simulink model "mainV02_43"  (R2016b)
settings: Solver=FixedStepAuto  StartTime=0.0  StopTime=inf  FixedStep=Ts  MaxStep=0.2  RelTol=1e-2
undefined symbols (not defined in the file): checks, decyear, deltae_degrees, deltafl_degrees, deltafr_degrees, deltar_degrees, deltat_1, deltat_2, deltat_3, deltat_4, deltat_5, Earth, F, ft, groundReaction, initDate, initialValues, LD, leapyear, Light, m, MIL, Newton, Raphson, s, sigbuilder_block, Ts, Vehicle, WGS84
libraries: simulink x21, aerolibutil x19, aerolibtransform2 x9, aerolib6dofsys x5, aerolibasang x4, aerolib6dof2 x4, aerolibwind2 x3, aerolibbdyn x3, aerolibconvert2 x3, aerolibactuator x2, aerolibgravity2 x2, aerolibnav x2
(part 3 of 6)

== system mainV02_43/LIBIS Plant/Custom Variable Mass 6DOF (Euler Angles) (propio) ==
  Forces : Inport  Unit=N  PortDimensions=3
  Moments : Inport  Port=2  Unit=N*m  PortDimensions=3
  m_dot : Inport  Port=3  Unit=kg/s
  mass : Inport  Port=4  Unit=kg
  I_dot : Inport  Port=5  Unit=kg*m^2/s  PortDimensions=[3 3]
  I : Inport  Port=6  Unit=kg*m^2  PortDimensions=[3 3]
  Vre : Inport  Port=7  Unit=m/s
  Calculate DCM & Euler Angles : aerolib6dofsys/DCM & Euler Angles (Euler)  SystemSampleTime=-1
  Calculate omega_dot : aerolib6dofsys/Calculate omega_dot  SystemSampleTime=-1
  "Determine Force, Mass & Inertia" : aerolib6dofsys/Mass & Inertia (custom)  SystemSampleTime=-1
  Disallow CGS : UnitConfiguration  UnitSystemsStr=English,SI,SI (extended)  AllowAllUnitSystems=off
  Out9 : Terminator
  Product : Product  Inputs=*/  SaturateOnIntegerOverflow=on  OutDataTypeStr=Inherit: Same as first input
  Reshape : Reshape  OutputDimensions=""
  Sum2 : Sum  Inputs=|++  SaturateOnIntegerOverflow=on
  Transpose : Math  Operator=transpose  SaturateOnIntegerOverflow=on
  Vbxw : aerolibutil/3x3 Cross Product
  Velocity Conversion : aerolib6dof2/6DOF (Euler Angles)/Velocity Conversion
  Velocity Conversion1 : aerolib6dof2/6DOF (Euler Angles)/Velocity Conversion1
  Velocity Conversion2 : aerolib6dof2/6DOF (Euler Angles)/Velocity Conversion2
  "p,q,r " : Integrator  InitialCondition=pm_0
  "transform to Inertial axes " : aerolib6dof2/6DOF (Euler Angles)/transform to Inertial axes   SystemSampleTime=-1
  ub,vb,wb : Integrator  InitialCondition=Vm_0
  xe,ye,ze : Integrator  InitialCondition=xme_0  UpperSaturationLimit=[inf, inf, initialValues.href]  LowerSaturationLimit=[-inf, -inf, -inf]
  Ve : Outport  Unit=m/s
  Xe : Outport  Port=2  Unit=m
  Euler : Outport  Port=3  Unit=rad
  DCM : Outport  Port=4  Unit=1
  Vb : Outport  Port=5  Unit=m/s
  p,q,r : Outport  Port=6  Unit=rad/s
  pdot,qdot,rdot : Outport  Port=7  Unit=rad/s^2
  Ab : Outport  Port=8  Unit=m/s^2  PortDimensions=3
  wires:
  Velocity Conversion1/1 -> Ve/1
  "Determine Force, Mass & Inertia"/2 -> Product/2
  Vre/1 -> Velocity Conversion2/1
  Calculate DCM & Euler Angles/1 -> DCM/1, Transpose/1
  Transpose/1 -> "transform to Inertial axes "/2
  Calculate DCM & Euler Angles/2 -> Euler/1
  "Determine Force, Mass & Inertia"/4 -> Out9/1
  "p,q,r "/1 -> Calculate DCM & Euler Angles/1, p,q,r/1, Vbxw/2, Calculate omega_dot/1
  xe,ye,ze/1 -> Xe/1
  Velocity Conversion/1 -> Vb/1
  I_dot/1 -> "Determine Force, Mass & Inertia"/6
  "transform to Inertial axes "/1 -> Velocity Conversion1/1, xe,ye,ze/1
  mass/1 -> "Determine Force, Mass & Inertia"/3
  Velocity Conversion2/1 -> "Determine Force, Mass & Inertia"/1
  "Determine Force, Mass & Inertia"/1 -> Product/1
  Forces/1 -> "Determine Force, Mass & Inertia"/2
  Moments/1 -> Calculate omega_dot/3
  Product/1 -> Sum2/1
  m_dot/1 -> "Determine Force, Mass & Inertia"/4
  ub,vb,wb/1 -> Vbxw/1, "transform to Inertial axes "/1, Velocity Conversion/1
  "Determine Force, Mass & Inertia"/3 -> Calculate omega_dot/2
  I/1 -> "Determine Force, Mass & Inertia"/5
  Sum2/1 -> Ab/1, ub,vb,wb/1
  Calculate omega_dot/1 -> pdot,qdot,rdot/1, "p,q,r "/1
  Vbxw/1 -> Reshape/1
  Reshape/1 -> Sum2/2

== system mainV02_43/LIBIS Plant/Incidence, Sideslip ==
  "u, v, w" : Inport
  Airspeed : Sqrt  AlgorithmType=Newton-Raphson  SaturateOnIntegerOverflow=on
  Constant : Constant  Value=0
  Incidence : Trigonometry  Operator=atan2
  Product : Product  Inputs=*/  SaturateOnIntegerOverflow=on  OutDataTypeStr=Inherit: Same as first input
  Sideslip : Trigonometry  Operator=asin
  Subsystem : aerolibasang/Incidence, Sideslip, & Airspeed/Subsystem
  Subsystem1 : aerolibasang/Incidence, Sideslip, & Airspeed/Subsystem1
  Switch : Switch  Criteria=u2 > Threshold
  dot : aerolibasang/Incidence, Sideslip, & Airspeed/dot
  Alpha : Outport  Unit=rad  InitialOutput=0
  Beta : Outport  Port=2  Unit=rad  InitialOutput=0
  wires:
  Subsystem/1 -> Incidence/1
  Subsystem1/1 -> Product/1
  dot/1 -> Airspeed/1
  Airspeed/1 -> Switch/2, Product/2
  "u, v, w"/1 -> Subsystem/1, Subsystem1/1, dot/1
  Sideslip/1 -> Beta/1
  Product/1 -> Switch/1
  Switch/1 -> Sideslip/1
  Constant/1 -> Switch/3
  Subsystem/2 -> Incidence/2
  Incidence/1 -> Alpha/1

== system mainV02_43/LIBIS Plant/Inertia Block ==
  Estimate Center of Gravity : aerolibbdyn/Estimate Center of Gravity  fmass=LD.Inertia.fullMass  emass=LD.Inertia.emptyMass-1  fcg=LD.Inertia.fullCG  ecg=LD.Inertia.emptyCG
  Ixx : Constant  Value=LD.Inertia.Ixx
  Ixy : Constant  Value=LD.Inertia.Ixy
  Ixz : Constant  Value=LD.Inertia.Ixz
  Iyy : Constant  Value=LD.Inertia.Iyy
  Iyz : Constant  Value=LD.Inertia.Iyz
  Izz : Constant  Value=LD.Inertia.Izz
  Mux : Mux  Inputs=3
  Reshape : Reshape
  Symmetric Inertia Tensor : aerolibbdyn/Symmetric Inertia Tensor
  Symmetric Inertia Tensor1 : aerolibbdyn/Symmetric Inertia Tensor
  Vre_x (m/s) : Constant  Value=LD.Inertia.dmassdxb
  Vre_y (m/s) : Constant  Value=LD.Inertia.dmassdyb
  Vre_z (m/s) : Constant  Value=LD.Inertia.dmassdzb
  dIxx/dt : Constant  Value=LD.Inertia.dIxx
  dIxy/dt : Constant  Value=LD.Inertia.dIxy
  dIxz/dt : Constant  Value=LD.Inertia.dIxz
  dIyy/dt : Constant  Value=LD.Inertia.dIyy
  dIyz/dt : Constant  Value=LD.Inertia.dIyz
  dIzz/dt : Constant  Value=LD.Inertia.dIzz
  dmass/dt (kg/s) : Constant  Value=LD.Inertia.dmass
  mass (kg) : Constant  Value=LD.Inertia.mass
  dm/dt (kg/s) : Outport  Unit=kg/s
  m (kg) : Outport  Port=2  Unit=kg
  dI/dt (kg-m^2/s) : Outport  Port=3  Unit=kg*meter^2/s
  I (kg-m^2) : Outport  Port=4  Unit=kg*meter*meter
  Vre (m/s) : Outport  Port=5  Unit=meter/s
  CG : Outport  Port=6
  dCG/dt : Outport  Port=7
  wires:
  Symmetric Inertia Tensor/1 -> I (kg-m^2)/1  "I (kg-m^2)"
  Symmetric Inertia Tensor1/1 -> dI/dt (kg-m^2/s)/1  "dI/dt (kg-m^2/s)"
  dIxx/dt/1 -> Symmetric Inertia Tensor1/1  "dIxx/dt (kg-m^2/s)"
  dIxz/dt/1 -> Symmetric Inertia Tensor1/3  "dIxz/dt (kg-m^2/s)"
  dIxy/dt/1 -> Symmetric Inertia Tensor1/2  "dIxy/dt (kg-m^2/s)"
  dIyy/dt/1 -> Symmetric Inertia Tensor1/4  "dIyy/dt (kg-m^2/s)"
  dIzz/dt/1 -> Symmetric Inertia Tensor1/6  "dIzz/dt (kg-m^2/s)"
  dIyz/dt/1 -> Symmetric Inertia Tensor1/5  "dIyz/dt (kg-m^2/s)"
  Ixx/1 -> Symmetric Inertia Tensor/1  "Ixx (kg-m^2)"
  Ixz/1 -> Symmetric Inertia Tensor/3  "Ixz (kg-m^2)"
  Ixy/1 -> Symmetric Inertia Tensor/2  "Ixy (kg-m^2)"
  Iyy/1 -> Symmetric Inertia Tensor/4  "Iyy (kg-m^2)"
  Izz/1 -> Symmetric Inertia Tensor/6  "Izz (kg-m^2)"
  Iyz/1 -> Symmetric Inertia Tensor/5  "Iyz (kg-m^2)"
  mass (kg)/1 -> Estimate Center of Gravity/1, m (kg)/1  "m (kg)"
  dmass/dt (kg/s)/1 -> Estimate Center of Gravity/2, dm/dt (kg/s)/1  "dm/dt (kg/s)"
  Vre_x (m/s)/1 -> Mux/1  "Vre_x (m/s)"
  Vre_z (m/s)/1 -> Mux/3  "Vre_z (m/s)"
  Vre_y (m/s)/1 -> Mux/2  "Vre_y (m/s)"
  Mux/1 -> Vre (m/s)/1  "Vre (m/s)"
  Estimate Center of Gravity/1 -> Reshape/1  "CG"
  Estimate Center of Gravity/2 -> dCG/dt/1  "dCG/dt"
  Reshape/1 -> CG/1

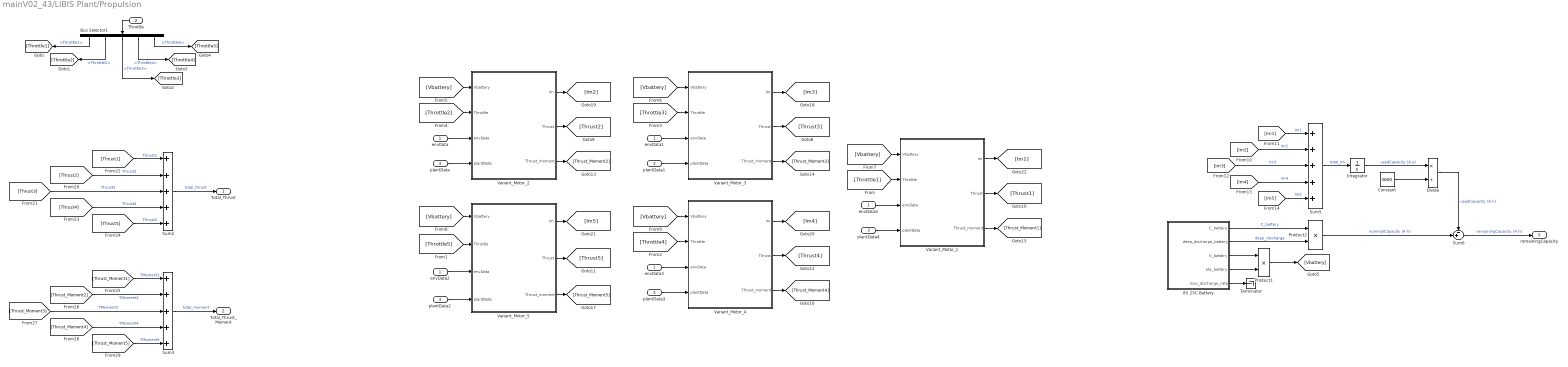
== system mainV02_43/LIBIS Plant/Propulsion ==
  envData : Inport
  Throttle : Inport  Port=2
  plantData : Inport  Port=3
  8S 25C Battery : Subsystem
  Bus Selector1 : BusSelector  OutputSignals=Throttle1,Throttle2,Throttle3,Throttle4,Throttle5
  Constant : Constant  Value=3600
  Divide : Product  Inputs=*/
  Integrator : Integrator
  Product1 : Product
  Product2 : Product
  Sum2 : Sum  Inputs=+++++
  Sum3 : Sum  Inputs=+++++
  Sum5 : Sum  Inputs=+++++
  Sum6 : Sum  Inputs=-+|
  Terminator : Terminator
  Variant_Motor_1 : Subsystem  Variant=on
      mask Display:
      | imageName='LIBIS_Motor1.png';
      | currentPath=get_param(bdroot, 'FileName');
      | positions=strfind(currentPath,'\');
      | imagePath=strcat(currentPath(1:positions(end-1)),'graphics\',imageName);
      | image(imagePath);
  Variant_Motor_2 : Subsystem  Variant=on
      mask Display:
      | imageName='LIBIS_Motor2.png';
      | currentPath=get_param(bdroot, 'FileName');
      | positions=strfind(currentPath,'\');
      | imagePath=strcat(currentPath(1:positions(end-1)),'graphics\',imageName);
      | image(imagePath);
  Variant_Motor_3 : Subsystem  Variant=on
      mask Display:
      | imageName='LIBIS_Motor3.png';
      | currentPath=get_param(bdroot, 'FileName');
      | positions=strfind(currentPath,'\');
      | imagePath=strcat(currentPath(1:positions(end-1)),'graphics\',imageName);
      | image(imagePath);
  Variant_Motor_4 : Subsystem  Variant=on
      mask Display:
      | imageName='LIBIS_Motor4.png';
      | currentPath=get_param(bdroot, 'FileName');
      | positions=strfind(currentPath,'\');
      | imagePath=strcat(currentPath(1:positions(end-1)),'graphics\',imageName);
      | image(imagePath);
  Variant_Motor_5 : Subsystem  Variant=on
      mask Display:
      | imageName='LIBIS_Motor5.png';
      | currentPath=get_param(bdroot, 'FileName');
      | positions=strfind(currentPath,'\');
      | imagePath=strcat(currentPath(1:positions(end-1)),'graphics\',imageName);
      | image(imagePath);
  envData{1..4} (4 alike) : InportShadow
  plantData{1..4} (4 alike) : InportShadow  Port=3
  Total_Thrust : Outport
  Total_Thrust_Moment : Outport  Port=2
  remainingCapacity : Outport  Port=3
  wires:
  Throttle/1 -> Bus Selector1/1
  Bus Selector1/1 -> [Throttle1]  "<Throttle1>"
  Bus Selector1/2 -> [Throttle2]  "<Throttle2>"
  Bus Selector1/3 -> [Throttle3]  "<Throttle3>"
  Bus Selector1/4 -> [Throttle4]  "<Throttle4>"
  Bus Selector1/5 -> [Throttle5]  "<Throttle5>"
  8S 25C Battery/3(V_battery) -> Product1/1
  8S 25C Battery/4(eta_battery) -> Product1/2
  8S 25C Battery/1(C_battery) -> Product2/1  "C_battery"
  8S 25C Battery/5(max_discharge_rate) -> Terminator/1
  8S 25C Battery/2(deep_discharge_battery) -> Product2/2  "deep_discharge"
  [Throttle5] -> Variant_Motor_5/2(Throttle)
  Variant_Motor_5/2(Thrust) -> [Thrust5]
  [Thrust1] -> Sum2/1  "Thrust1"
  [Thrust2] -> Sum2/2  "Thrust2"
  [Thrust3] -> Sum2/3  "Thrust3"
  [Thrust4] -> Sum2/4  "Thrust4"
  [Thrust5] -> Sum2/5  "Thrust5"
  Sum2/1 -> Total_Thrust/1  "total_thrust"
  Sum3/1 -> Total_Thrust_Moment/1  "total_moment"
  [Thrust_Moment1] -> Sum3/1  "TMoment1"
  [Thrust_Moment2] -> Sum3/2  "TMoment2"
  [Thrust_Moment3] -> Sum3/3  "TMoment3"
  [Thrust_Moment4] -> Sum3/4  "TMoment4"
  Variant_Motor_5/3(Thrust_moment) -> [Thrust_Moment5]
  [Thrust_Moment5] -> Sum3/5  "TMoment5"
  Product2/1 -> Sum6/2  "nominalCapacity (A·h)"
  Variant_Motor_5/1(Im) -> [Im5]
  [Im3] -> Sum5/3  "Im3"
  [Im2] -> Sum5/2  "Im2"
  [Im1] -> Sum5/1  "Im1"
  [Im4] -> Sum5/4  "Im4"
  [Im5] -> Sum5/5  "Im5"
  Sum5/1 -> Integrator/1  "total_Im"
  Sum6/1 -> remainingCapacity/1  "remainingCapacity (A·h)"
  Product1/1 -> [Vbattery]
  [Vbattery] -> Variant_Motor_5/1(Vbattery)
  Integrator/1 -> Divide/1  "usedCapacity (A·s)"
  Constant/1 -> Divide/2
  Divide/1 -> Sum6/1  "usedCapacity (A·h)"
  envData2/1 -> Variant_Motor_5/3(envData)
  plantData2/1 -> Variant_Motor_5/4(plantData)
  [Vbattery] -> Variant_Motor_2/1(Vbattery)
  [Throttle2] -> Variant_Motor_2/2(Throttle)
  Variant_Motor_2/1(Im) -> [Im2]
  Variant_Motor_2/2(Thrust) -> [Thrust2]
  Variant_Motor_2/3(Thrust_moment) -> [Thrust_Moment2]
  envData/1 -> Variant_Motor_2/3(envData)
  plantData/1 -> Variant_Motor_2/4(plantData)
  [Vbattery] -> Variant_Motor_3/1(Vbattery)
  [Throttle3] -> Variant_Motor_3/2(Throttle)
  Variant_Motor_3/3(Thrust_moment) -> [Thrust_Moment3]
  Variant_Motor_3/2(Thrust) -> [Thrust3]
  Variant_Motor_3/1(Im) -> [Im3]
  envData1/1 -> Variant_Motor_3/3(envData)
  plantData1/1 -> Variant_Motor_3/4(plantData)
  [Vbattery] -> Variant_Motor_4/1(Vbattery)
  [Throttle4] -> Variant_Motor_4/2(Throttle)
  Variant_Motor_4/1(Im) -> [Im4]
  Variant_Motor_4/2(Thrust) -> [Thrust4]
  Variant_Motor_4/3(Thrust_moment) -> [Thrust_Moment4]
  envData3/1 -> Variant_Motor_4/3(envData)
  plantData3/1 -> Variant_Motor_4/4(plantData)
  [Vbattery] -> Variant_Motor_1/1(Vbattery)
  [Throttle1] -> Variant_Motor_1/2(Throttle)
  Variant_Motor_1/1(Im) -> [Im1]
  Variant_Motor_1/2(Thrust) -> [Thrust1]
  Variant_Motor_1/3(Thrust_moment) -> [Thrust_Moment1]
  envData4/1 -> Variant_Motor_1/3(envData)
  plantData4/1 -> Variant_Motor_1/4(plantData)

== system mainV02_43/LIBIS Plant/Subsystem ==
  beta : Inport  Unit=rad
  alpha : Inport  Port=2  Unit=rad
  V_body : Inport  Port=3  Unit=meter/s
  Omega_body : Inport  Port=4  Unit=rad/s
  Accel_body : Inport  Port=5  Unit=m/s^2
  Constant1 : Constant  Value=0
  Constant11 : Constant  Value=0
  Direction Cosine Matrix Body to Wind : aerolibtransform2/Direction Cosine Matrix Body to Wind
  IC : InitialCondition  Value=0
  Mux4 : Mux  Inputs=2
  Product1 : Product  Multiplication=Matrix(*)  SaturateOnIntegerOverflow=on  InputSameDT=on  OutDataTypeStr=Inherit: Same as first input
  Selector : Selector  InputPortWidth=3  IndexOptions=Index vector (dialog)  Indices=[2]  OutputSizes=1
  Terminator : Terminator
  calc alpha_dot : Subsystem
  alpha_dot : Outport  Unit=rad/s
  beta_dot : Outport  Port=2
  wires:
  Direction Cosine Matrix Body to Wind/1 -> Product1/1
  Product1/1 -> calc alpha_dot/4(Vw)
  Mux4/1 -> Direction Cosine Matrix Body to Wind/1, calc alpha_dot/2(alpha,beta)
  Constant11/1 -> beta_dot/1  "beta_dot"
  alpha/1 -> Mux4/1
  Omega_body/1 -> Selector/1
  V_body/1 -> Product1/2
  Accel_body/1 -> calc alpha_dot/3(Ab)
  beta/1 -> Mux4/2
  calc alpha_dot/1(alpha_dot) -> IC/1
  Selector/1 -> calc alpha_dot/1(q)  "q"
  IC/1 -> Terminator/1
  Constant1/1 -> alpha_dot/1

== system mainV02_43/LIBIS Plant/TransferFunction ==
  In1 : Inport
  Demux4 : Demux  Outputs=3
  Mux1 : Mux  Inputs=3
  Transfer Fcn1 : TransferFcn  Denominator=[eps 1]
  Transfer Fcn4 : TransferFcn  Denominator=[eps 1]
  Transfer Fcn5 : TransferFcn  Denominator=[eps 1]
  Out1 : Outport
  wires:
  Transfer Fcn1/1 -> Mux1/1
  Transfer Fcn5/1 -> Mux1/3
  Mux1/1 -> Out1/1
  Demux4/2 -> Transfer Fcn4/1
  Transfer Fcn4/1 -> Mux1/2
  Demux4/1 -> Transfer Fcn1/1
  In1/1 -> Demux4/1
  Demux4/3 -> Transfer Fcn5/1

== system mainV02_43/LIBIS Plant/TransferFunctions ==
  In1 : Inport
  In2 : Inport  Port=2
  Demux : Demux  Outputs=3
  Demux1 : Demux  Outputs=3
  Mux : Mux  Inputs=3
  Mux1 : Mux  Inputs=3
  Transfer Fcn{,1..5} (6 alike) : TransferFcn  Denominator=[eps 1]
  Out1 : Outport
  Out2 : Outport  Port=2
  wires:
  Demux1/3 -> Transfer Fcn5/1
  Transfer Fcn3/1 -> Mux1/1
  In2/1 -> Demux1/1
  Transfer Fcn1/1 -> Mux/2
  Demux1/2 -> Transfer Fcn4/1
  Demux/1 -> Transfer Fcn/1
  Transfer Fcn4/1 -> Mux1/2
  Transfer Fcn2/1 -> Mux/3
  Transfer Fcn5/1 -> Mux1/3
  Transfer Fcn/1 -> Mux/1
  Demux/3 -> Transfer Fcn2/1
  Demux/2 -> Transfer Fcn1/1
  Mux1/1 -> Out2/1
  Demux1/1 -> Transfer Fcn3/1
  In1/1 -> Demux/1
  Mux/1 -> Out1/1

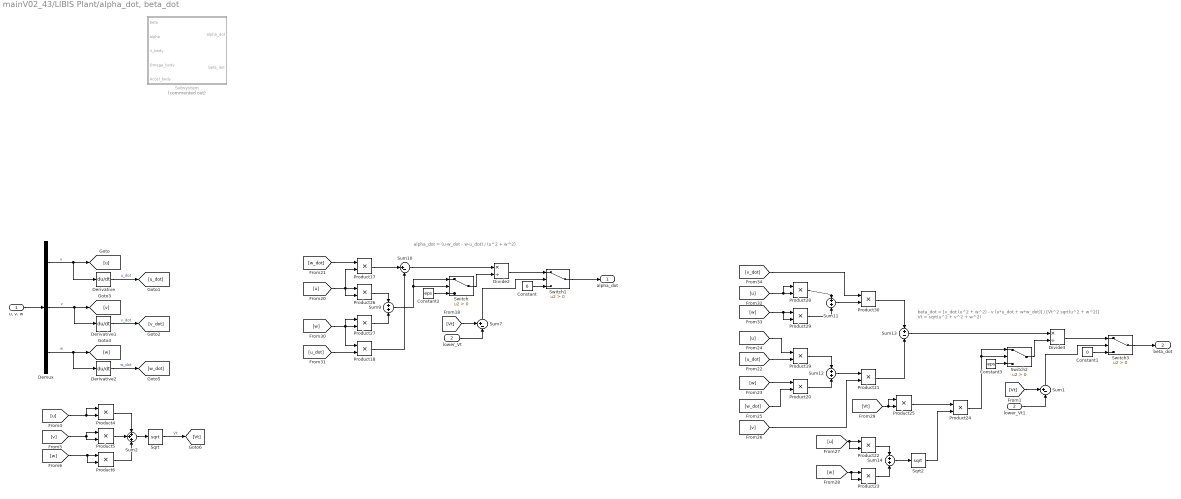
== system mainV02_43/LIBIS Plant/alpha_dot, beta_dot ==
  note: beta_dot = [v_dot (u^2 + w^2) - v (u*u_dot + w*w_dot)] / [Vt^2 sqrt(u^2 + w^2)]
      | Vt = sqrt(u^2 + v^2 + w^2)
  note: alpha_dot = (u·w_dot - w·u_dot) / (u^2 + w^2)
  "u, v, w" : Inport  Unit=meter/s
  lower_Vt : Inport  Port=2
  Constant : Constant  Value=0
  Constant1 : Constant  Value=0
  Constant2 : Constant  Value=eps
  Constant3 : Constant  Value=eps
  Demux : Demux  Outputs=3
  Derivative : Derivative
  Derivative1 : Derivative
  Derivative2 : Derivative
  Divide2 : Product  Inputs=*/
  Divide3 : Product  Inputs=*/
  Product{4..6,17..30} (17 alike) : Product
  Sqrt : Sqrt  SaturateOnIntegerOverflow=on
  Sqrt2 : Sqrt  SaturateOnIntegerOverflow=on
  Subsystem : Subsystem  Commented=on
  Sum1 : Sum  Inputs=+-|
  Sum10 : Sum  Inputs=|+-
  Sum{9,11..12,14} (4 alike) : Sum  Inputs=+|+
  Sum13 : Sum  Inputs=+|-
  Sum2 : Sum  Inputs=+++
  Sum7 : Sum  Inputs=+-|
  Switch{,1..3} (4 alike) : Switch  Criteria=u2 > Threshold
  lower_Vt1 : InportShadow  Port=2
  alpha_dot : Outport  Unit=rad/s
  beta_dot : Outport  Port=2
  wires:
  "u, v, w"/1 -> Demux/1
  Demux/1 -> Derivative/1, [u]  "u"
  Demux/2 -> Derivative1/1, [v]  "v"
  Demux/3 -> Derivative2/1, [w]  "w"
  [u] -> Product4/1, Product4/2
  [w] -> Product6/2, Product6/1
  [v] -> Product5/1, Product5/2
  Product4/1 -> Sum2/1
  Product6/1 -> Sum2/3
  Product5/1 -> Sum2/2
  Sum2/1 -> Sqrt/1
  Sqrt/1 -> [Vt]  "Vt"
  Derivative2/1 -> [w_dot]  "w_dot"
  Derivative/1 -> [u_dot]  "u_dot"
  Derivative1/1 -> [v_dot]  "v_dot"
  Sum7/1 -> Switch1/2
  [Vt] -> Sum7/1
  lower_Vt/1 -> Sum7/2
  [w_dot] -> Product17/1
  [u] -> Product17/2, Product26/2, Product26/1
  [w] -> Product27/1, Product27/2, Product18/1
  [u_dot] -> Product18/2
  Product26/1 -> Sum9/1
  Product27/1 -> Sum9/2
  Product17/1 -> Sum10/1
  Product18/1 -> Sum10/2
  Sum10/1 -> Divide2/1
  [u] -> Product28/1, Product28/2
  [w] -> Product29/2, Product29/1
  Product28/1 -> Sum11/1
  Product29/1 -> Sum11/2
  Sum11/1 -> Product30/2
  [v_dot] -> Product30/1
  [u_dot] -> Product19/2
  [w] -> Product20/1
  Product19/1 -> Sum12/1
  Product20/1 -> Sum12/2
  Sum12/1 -> Product21/1
  [u] -> Product19/1
  [w_dot] -> Product20/2
  [v] -> Product21/2
  Product30/1 -> Sum13/1
  Product21/1 -> Sum13/2
  Sum13/1 -> Divide3/1
  Product22/1 -> Sum14/1
  Product23/1 -> Sum14/2
  [u] -> Product22/2, Product22/1
  [w] -> Product23/2, Product23/1
  [Vt] -> Product25/1, Product25/2
  Product25/1 -> Product24/1
  Sum14/1 -> Sqrt2/1
  Sqrt2/1 -> Product24/2
  Switch/1 -> Divide2/2
  Sum9/1 -> Switch/2, Switch/1
  Constant2/1 -> Switch/3
  Switch2/1 -> Divide3/2
  Product24/1 -> Switch2/2, Switch2/1
  Constant3/1 -> Switch2/3
  Switch3/1 -> beta_dot/1
  Divide2/1 -> Switch1/1
  Switch1/1 -> alpha_dot/1
  Constant/1 -> Switch1/3
  Sum1/1 -> Switch3/2
  Constant1/1 -> Switch3/3
  Divide3/1 -> Switch3/1
  [Vt] -> Sum1/1
  lower_Vt1/1 -> Sum1/2

== system mainV02_43/Pilot Commands/Signal Builder ==
  Demux : Demux  Tag=STV Demux  Outputs=9
  FromWs : FromWorkspace  Tag=STV FromWs  VariableName=tuvar  SampleTime=0
      SigBuilderData=|
      | common.afterFinalStr = 'Extrapolate'
      | common.sampleTime = 0
      | dataSet.timeRange = [0 500]
      | dataSet.name = 'Group 1'
      | sbobj.Groups.Name = 'Group 1'
      | sbobj.Groups.Signals(1).Name = 'Roll'
      | sbobj.Groups.Signals(1).XData = [0 500]
      | sbobj.Groups.Signals(1).YData = [0 0]
      | sbobj.Groups.Signals(2).Name = 'Pitch'
      | sbobj.Groups.Signals(2).XData = [0 500]
      | sbobj.Groups.Signals(2).YData = [0 0]
      | sbobj.Groups.Signals(3).Name = 'Yaw'
      | sbobj.Groups.Signals(3).XData = [0 500]
      | sbobj.Groups.Signals(3).YData = [0 0]
      | sbobj.Groups.Signals(4).Name = 'Altitude'
      | sbobj.Groups.Signals(4).XData = [0 50 50 200 200 300 300 500]
      | sbobj.Groups.Signals(4).YData = [0 0 100 100 200 200 0 0]
      | sbobj.Groups.Signals(5).Name = 'Throttle1'
      | sbobj.Groups.Signals(5).XData = [0 500]
      | sbobj.Groups.Signals(5).YData = [0 0]
      | sbobj.Groups.Signals(6).Name = 'Throttle2'
      | sbobj.Groups.Signals(6).XData = [0 500]
      | sbobj.Groups.Signals(6).YData = [0 0]
      | sbobj.Groups.Signals(7).Name = 'Throttle3'
      | sbobj.Groups.Signals(7).XData = [0 500]
      | sbobj.Groups.Signals(7).YData = [0 0]
      | sbobj.Groups.Signals(8).Name = 'Throttle4'
      | sbobj.Groups.Signals(8).XData = [0 500]
      | sbobj.Groups.Signals(8).YData = [0 0]
      | sbobj.Groups.Signals(9).Name = 'Throttle5'
      | sbobj.Groups.Signals(9).XData = [0 500]
      | sbobj.Groups.Signals(9).YData = [0 0]
      | sbobj.Groups.TimeRange = [0 500]
  Roll : Outport  Tag=STV Outport
  Pitch : Outport  Tag=STV Outport  Port=2
  Yaw : Outport  Tag=STV Outport  Port=3
  Altitude : Outport  Tag=STV Outport  Port=4
  Throttle1 : Outport  Tag=STV Outport  Port=5
  Throttle2 : Outport  Tag=STV Outport  Port=6
  Throttle3 : Outport  Tag=STV Outport  Port=7
  Throttle4 : Outport  Tag=STV Outport  Port=8
  Throttle5 : Outport  Tag=STV Outport  Port=9
  wires:
  FromWs/1 -> Demux/1
  Demux/1 -> Roll/1
  Demux/2 -> Pitch/1
  Demux/3 -> Yaw/1
  Demux/4 -> Altitude/1
  Demux/5 -> Throttle1/1
  Demux/6 -> Throttle2/1
  Demux/7 -> Throttle3/1
  Demux/8 -> Throttle4/1
  Demux/9 -> Throttle5/1

== system mainV02_43/Sensors/Feedthrough Sensors ==
  States : Inport  OutDataTypeStr=Bus: plantDataBus
  Environment : Inport  Port=2  OutDataTypeStr=Bus: envDataBus
  Bus Creator2 : BusCreator  Inputs='LLAMeas','X_nedMeas','VearthMeas','AccelMeas_body','OmegaMeas_body','DCMMeas_body_earth','EulerMeas','VaeroMeas_body','alphaMeas','betaMeas','CGMeas','remainingCapacityMeas'  OutDataTypeStr=Bus: SensorsBus  NonVirtualBus=on
  CPU : Subsystem
  Environment_1 : InportShadow  Port=2  OutDataTypeStr=Bus: envDataBus
  GPS : Subsystem
  IMU : Subsystem
  Pitot : Subsystem
  Veleta : Subsystem
  Sensors : Outport  OutDataTypeStr=Bus: SensorsBus
  wires:
  Environment/1 -> IMU/2(Environment)
  IMU/4(EulerMeas) -> Bus Creator2/7  "EulerMeas"
  Bus Creator2/1 -> Sensors/1  "Sensors"
  CPU/1(CGMeas) -> Bus Creator2/11  "CGMeas"
  GPS/2(X_nedMeas) -> Bus Creator2/2  "X_nedMeas"
  States/1 -> IMU/1(States), GPS/1(States), Pitot/1(States), CPU/1(States), Veleta/1(States)
  IMU/2(OmegaMeas_body) -> Bus Creator2/5  "OmegaMeas_body"
  IMU/1(AccelMeas_body) -> Bus Creator2/4  "AccelMeas_body"
  GPS/1(LLAMeas) -> Bus Creator2/1  "LLAMeas"
  Veleta/1(alphaMeas) -> Bus Creator2/9  "alphaMeas"
  Environment_1/1 -> Pitot/2(Environment)
  Veleta/2(betaMeas) -> Bus Creator2/10  "betaMeas"
  Pitot/1(VaeroMeas_body) -> Bus Creator2/8  "VaeroMeas_body"
  CPU/2(remainingCapacityMeas) -> Bus Creator2/12  "remainingCapacityMeas"
  GPS/3(VearthMeas) -> Bus Creator2/3  "VearthMeas"
  IMU/3(DCMMeas_body_earth) -> Bus Creator2/6  "DCMMeas_body_earth"

== system mainV02_43/Sensors/Noisy Sensors ==
  States : Inport  OutDataTypeStr=Bus: plantDataBus
  Environment : Inport  Port=2  OutDataTypeStr=Bus: envDataBus
  Bus Creator2 : BusCreator  Inputs='LLAMeas','X_nedMeas','VearthMeas','AccelMeas_body','OmegaMeas_body','DCMMeas_body_earth','EulerMeas','VaeroMeas_body','alphaMeas','betaMeas','CGMeas','remainingCapacityMeas'  OutDataTypeStr=Bus: SensorsBus  NonVirtualBus=on
  CPU (Feedthough) : Subsystem
  Environment_1 : InportShadow  Port=2  OutDataTypeStr=Bus: envDataBus
  GPS (Feedthough) : Subsystem
  IMU : Subsystem
  Pitot (Feedthough) : Subsystem
  Veleta (Feedthough) : Subsystem
  Sensors : Outport  OutDataTypeStr=Bus: SensorsBus
  wires:
  Environment/1 -> IMU/2(Environment)
  IMU/4(EulerMeas) -> Bus Creator2/7  "EulerMeas"
  Bus Creator2/1 -> Sensors/1  "Sensors"
  CPU (Feedthough)/1(CGMeas) -> Bus Creator2/11  "CGMeas"
  GPS (Feedthough)/2(X_nedMeas) -> Bus Creator2/2  "X_nedMeas"
  States/1 -> GPS (Feedthough)/1(States), IMU/1(States), Pitot (Feedthough)/1(States), CPU (Feedthough)/1(States), Veleta (Feedthough)/1(States)
  IMU/2(OmegaMeas_body) -> Bus Creator2/5  "OmegaMeas_body"
  IMU/1(AccelMeas_body) -> Bus Creator2/4  "AccelMeas_body"
  GPS (Feedthough)/1(LLAMeas) -> Bus Creator2/1  "LLAMeas"
  Veleta (Feedthough)/1(alphaMeas) -> Bus Creator2/9  "alphaMeas"
  Environment_1/1 -> Pitot (Feedthough)/2(Environment)
  Veleta (Feedthough)/2(betaMeas) -> Bus Creator2/10  "betaMeas"
  Pitot (Feedthough)/1(VaeroMeas_body) -> Bus Creator2/8  "VaeroMeas_body"
  CPU (Feedthough)/2(remainingCapacityMeas) -> Bus Creator2/12  "remainingCapacityMeas"
  GPS (Feedthough)/3(VearthMeas) -> Bus Creator2/3  "VearthMeas"
  IMU/3(DCMMeas_body_earth) -> Bus Creator2/6  "DCMMeas_body_earth"

== system mainV02_43/Visualization/Airspeed Indicator ==

== system mainV02_43/Visualization/Altimeter ==

== system mainV02_43/Visualization/Artificial Horizon ==

== system mainV02_43/Visualization/Axes to VR Axes ==
  Xe : Inport
  Concatenate : Concatenate  NumInputs=3
  Constant : Constant  Value=1.01
  Demux : Demux  Outputs=3
  Sum : Sum  Inputs=|++
  rad-->deg : Gain  Gain=-1  SaturateOnIntegerOverflow=on  OutDataTypeStr=Inherit: Same as input  ParamDataTypeStr=Inherit: Same as input
  rad-->deg1 : Gain  Gain=-1  SaturateOnIntegerOverflow=on  OutDataTypeStr=Inherit: Same as input  ParamDataTypeStr=Inherit: Same as input
  Xe VR : Outport
  wires:
  Xe/1 -> Demux/1
  Concatenate/1 -> Xe VR/1
  rad-->deg1/1 -> Concatenate/2
  rad-->deg/1 -> Concatenate/1
  Demux/1 -> Concatenate/3
  Demux/2 -> rad-->deg/1
  Constant/1 -> Sum/2
  Demux/3 -> Sum/1
  Sum/1 -> rad-->deg1/1

== system mainV02_43/Visualization/Climb Rate Indicator ==

== system mainV02_43/Visualization/Euler to VR ==
  Euler Angles : Inport
  Axis Angle Vector : Subsystem
  Constant : Constant  Value=pi/2
  Demux : Demux  Outputs=3
  Mux : Mux  Inputs=2
  Mux1 : Mux  Inputs=2
  Mux2 : Mux  Inputs=2
  Quaternion Multiplication (Pitch & Yaw) : aerolibutil/Quaternion Multiplication
  Quaternion Multiplication (Roll) : aerolibutil/Quaternion Multiplication
  Quaternion Normalization : Subsystem
  Quaternion Normalization1 : Subsystem
  Quaternion Normalization2 : Subsystem
  Sum : Sum  Inputs=|++
  Vr Pitch Axes : Constant  Value=[0 0 1]
  Vr Roll Axes : Constant  Value=[1 0 0]
  Vr Yaw Axes : Constant  Value=[0 -1 0]
  Axis Angle : Outport
  wires:
  Quaternion Multiplication (Roll)/1 -> Axis Angle Vector/1(e0)
  Quaternion Multiplication (Pitch & Yaw)/1 -> Quaternion Multiplication (Roll)/2
  Axis Angle Vector/1(e0_norm) -> Axis Angle/1
  Quaternion Normalization/1(e0_norm) -> Quaternion Multiplication (Roll)/1
  Quaternion Normalization2/1(e0_norm) -> Quaternion Multiplication (Pitch & Yaw)/1
  Quaternion Normalization1/1(e0_norm) -> Quaternion Multiplication (Pitch & Yaw)/2
  Mux2/1 -> Quaternion Normalization2/1(e0)
  Mux1/1 -> Quaternion Normalization1/1(e0)
  Mux/1 -> Quaternion Normalization/1(e0)
  Vr Yaw Axes/1 -> Mux2/2
  Demux/2 -> Mux1/1
  Vr Pitch Axes/1 -> Mux1/2
  Demux/1 -> Mux/1
  Vr Roll Axes/1 -> Mux/2
  Euler Angles/1 -> Demux/1
  Sum/1 -> Mux2/1
  Demux/3 -> Sum/1
  Constant/1 -> Sum/2

== system mainV02_43/Visualization/Half Gauge ==

== system mainV02_43/Visualization/Heading Indicator ==

== system mainV02_43/Visualization/Subsystem ==
  "X_ned " : Inport
  Euler_angles : Inport  Port=2
  V_body : Inport  Port=3
  V_ned : Inport  Port=4
  Angle Conversion : aerolibconvert2/Angle Conversion  IU=rad  OU=deg
  Angle Conversion1 : aerolibconvert2/Angle Conversion  IU=rad  OU=deg
  Climbrate : Selector  IndexMode=Zero-based  InputPortWidth=3  IndexOptions=Index vector (dialog)  Indices=2  OutputSizes=1
  Concatenate : Concatenate
  Dot Product : DotProduct  SaturateOnIntegerOverflow=on  OutDataTypeStr=Inherit: Inherit via internal rule
  Flightpath Angle : Subsystem
  Heading : Selector  IndexMode=Zero-based  InputPortWidth=3  IndexOptions=Index vector (dialog)  Indices=2  OutputSizes=1
  Height : Selector  IndexMode=Zero-based  InputPortWidth=3  IndexOptions=Index vector (dialog)  Indices=2  OutputSizes=1
  Length Conversion : aerolibconvert2/Length Conversion  IU=m  OU=ft
  Roll Angle : Selector  IndexMode=Zero-based  InputPortWidth=3  IndexOptions=Index vector (dialog)  Indices=0  OutputSizes=1
  Velocity Conversion : aerolibconvert/Velocity Conversion  IU=m/s  OU=kts
  Velocity Conversion1 : aerolibconvert/Velocity Conversion  IU=m/s  OU=ft/s
  rad-->deg1 : Gain  Gain=-1  SaturateOnIntegerOverflow=on  OutDataTypeStr=Inherit: Same as input  ParamDataTypeStr=Inherit: Same as input
  rad-->deg2 : Gain  Gain=-1  SaturateOnIntegerOverflow=on  OutDataTypeStr=Inherit: Same as input  ParamDataTypeStr=Inherit: Same as input
  rad-->deg3 : Gain  Gain=60  SaturateOnIntegerOverflow=on  OutDataTypeStr=Inherit: Same as input  ParamDataTypeStr=Inherit: Same as input
  vt : Sqrt  SaturateOnIntegerOverflow=on
  Airspeed (kts) : Outport
  Height (ft) : Outport  Port=2
  Roll Flightpath (deg) : Outport  Port=3
  Climb Rate (ft/min) : Outport  Port=4
  Heading (deg) : Outport  Port=5
  wires:
  Velocity Conversion1/1 -> rad-->deg3/1
  rad-->deg3/1 -> Climb Rate (ft/min)/1
  V_ned/1 -> Flightpath Angle/1(Ve), Climbrate/1
  Flightpath Angle/1(gamma) -> Concatenate/2
  rad-->deg2/1 -> Velocity Conversion1/1
  Length Conversion/1 -> Height (ft)/1
  Angle Conversion1/1 -> Roll Flightpath (deg)/1
  Height/1 -> rad-->deg1/1
  Angle Conversion/1 -> Heading (deg)/1  "Heading"
  Heading/1 -> Angle Conversion/1
  Velocity Conversion/1 -> Airspeed (kts)/1
  Dot Product/1 -> vt/1
  Roll Angle/1 -> Concatenate/1
  V_body/1 -> Dot Product/2, Dot Product/1
  Concatenate/1 -> Angle Conversion1/1
  vt/1 -> Velocity Conversion/1
  Climbrate/1 -> rad-->deg2/1
  rad-->deg1/1 -> Length Conversion/1
  Euler_angles/1 -> Roll Angle/1, Heading/1
  "X_ned "/1 -> Height/1

== system mainV02_43/Environment/Terrain/Reaction ==
  X : Inport
  V : Inport  Port=2
  -D1 : Gain  Gain=-groundReaction.D
  -K2 : Gain  Gain=-groundReaction.K
  Constant3 : Constant  Value=0
  Constant4 : Constant  Value=0
  Constant5 : Constant  Value=0
  Mux1 : Mux  Inputs=3
  Product1 : Product
  Sel5 : Selector  InputPortWidth=3  IndexOptions=Index vector (dialog)  Indices=3  OutputSizes=1
  Sel6 : Selector  InputPortWidth=3  IndexOptions=Index vector (dialog)  Indices=3  OutputSizes=1
  Sqrt1 : Sqrt  SaturateOnIntegerOverflow=on
  Sum4 : Sum  Inputs=|++
  Sum5 : Sum  Inputs=-+
  Switch3 : Switch  Criteria=u2 > Threshold
  Ze2height1 : UnaryMinus
  Ze_dot2height_dot3 : UnaryMinus
  height2d2 : UnaryMinus
  height2d3 : UnaryMinus
  hground_value1 : Constant  Value=initialValues.href  OutDataTypeStr=double
  hground1 : Outport  Unit=m
  F_earth : Outport  Port=2
  wires:
  Ze2height1/1 -> Sum5/2  "alt"
  X/1 -> Sel6/1
  Sel6/1 -> Ze2height1/1
  Sel5/1 -> Ze_dot2height_dot3/1
  hground_value1/1 -> Sum5/1
  Constant3/1 -> Switch3/1
  Switch3/1 -> height2d2/1
  height2d2/1 -> Sqrt1/1  "d"
  -K2/1 -> Sum4/1
  Product1/1 -> height2d3/1
  height2d3/1 -> Mux1/3
  Sum5/1 -> hground1/1, -K2/1, Switch3/3, Switch3/2  "z"
  Sqrt1/1 -> Product1/1
  Ze_dot2height_dot3/1 -> -D1/1  "z_dot"
  -D1/1 -> Sum4/2
  Sum4/1 -> Product1/2
  V/1 -> Sel5/1
  Mux1/1 -> F_earth/1  "F_earth"
  Constant5/1 -> Mux1/2
  Constant4/1 -> Mux1/1

== system mainV02_43/Environment/Terrain/Reaction1 ==
  X : Inport
  V : Inport  Port=2
  -D1 : Gain  Gain=-groundReaction.D
  -K2 : Gain  Gain=-groundReaction.K
  Constant3 : Constant  Value=0
  Constant4 : Constant  Value=0
  Constant5 : Constant  Value=0
  Mux1 : Mux  Inputs=3
  Product1 : Product
  Sel5 : Selector  InputPortWidth=3  IndexOptions=Index vector (dialog)  Indices=3  OutputSizes=1
  Sel6 : Selector  InputPortWidth=3  IndexOptions=Index vector (dialog)  Indices=3  OutputSizes=1
  Sqrt1 : Sqrt  SaturateOnIntegerOverflow=on
  Sum4 : Sum  Inputs=|++
  Sum5 : Sum  Inputs=-+
  Switch3 : Switch  Criteria=u2 > Threshold
  Ze2height1 : UnaryMinus
  Ze_dot2height_dot3 : UnaryMinus
  height2d2 : UnaryMinus
  height2d3 : UnaryMinus
  hground_value1 : Constant  Value=initialValues.href  OutDataTypeStr=double
  hground1 : Outport  Unit=m
  F_earth : Outport  Port=2
  wires:
  Ze2height1/1 -> Sum5/2  "alt"
  X/1 -> Sel6/1
  Sel6/1 -> Ze2height1/1
  Sel5/1 -> Ze_dot2height_dot3/1
  hground_value1/1 -> Sum5/1
  Constant3/1 -> Switch3/1
  Switch3/1 -> height2d2/1
  height2d2/1 -> Sqrt1/1  "d"
  -K2/1 -> Sum4/1
  Product1/1 -> height2d3/1
  height2d3/1 -> Mux1/3
  Sum5/1 -> hground1/1, -K2/1, Switch3/3, Switch3/2  "z"
  Sqrt1/1 -> Product1/1
  Ze_dot2height_dot3/1 -> -D1/1  "z_dot"
  -D1/1 -> Sum4/2
  Sum4/1 -> Product1/2
  V/1 -> Sel5/1
  Mux1/1 -> F_earth/1  "F_earth"
  Constant5/1 -> Mux1/2
  Constant4/1 -> Mux1/1

== system mainV02_43/Environment/Terrain/Reaction2 ==
  X : Inport
  V : Inport  Port=2
  -D1 : Gain  Gain=-groundReaction.D
  -K2 : Gain  Gain=-groundReaction.K
  Constant3 : Constant  Value=0
  Constant4 : Constant  Value=0
  Constant5 : Constant  Value=0
  Mux1 : Mux  Inputs=3
  Product1 : Product
  Sel5 : Selector  InputPortWidth=3  IndexOptions=Index vector (dialog)  Indices=3  OutputSizes=1
  Sel6 : Selector  InputPortWidth=3  IndexOptions=Index vector (dialog)  Indices=3  OutputSizes=1
  Sqrt1 : Sqrt  SaturateOnIntegerOverflow=on
  Sum4 : Sum  Inputs=|++
  Sum5 : Sum  Inputs=-+
  Switch3 : Switch  Criteria=u2 > Threshold
  Ze2height1 : UnaryMinus
  Ze_dot2height_dot3 : UnaryMinus
  height2d2 : UnaryMinus
  height2d3 : UnaryMinus
  hground_value1 : Constant  Value=initialValues.href  OutDataTypeStr=double
  hground1 : Outport  Unit=m
  F_earth : Outport  Port=2
  wires:
  Ze2height1/1 -> Sum5/2  "alt"
  X/1 -> Sel6/1
  Sel6/1 -> Ze2height1/1
  Sel5/1 -> Ze_dot2height_dot3/1
  hground_value1/1 -> Sum5/1
  Constant3/1 -> Switch3/1
  Switch3/1 -> height2d2/1
  height2d2/1 -> Sqrt1/1  "d"
  -K2/1 -> Sum4/1
  Product1/1 -> height2d3/1
  height2d3/1 -> Mux1/3
  Sum5/1 -> hground1/1, -K2/1, Switch3/3, Switch3/2  "z"
  Sqrt1/1 -> Product1/1
  Ze_dot2height_dot3/1 -> -D1/1  "z_dot"
  -D1/1 -> Sum4/2
  Sum4/1 -> Product1/2
  V/1 -> Sel5/1
  Mux1/1 -> F_earth/1  "F_earth"
  Constant5/1 -> Mux1/2
  Constant4/1 -> Mux1/1

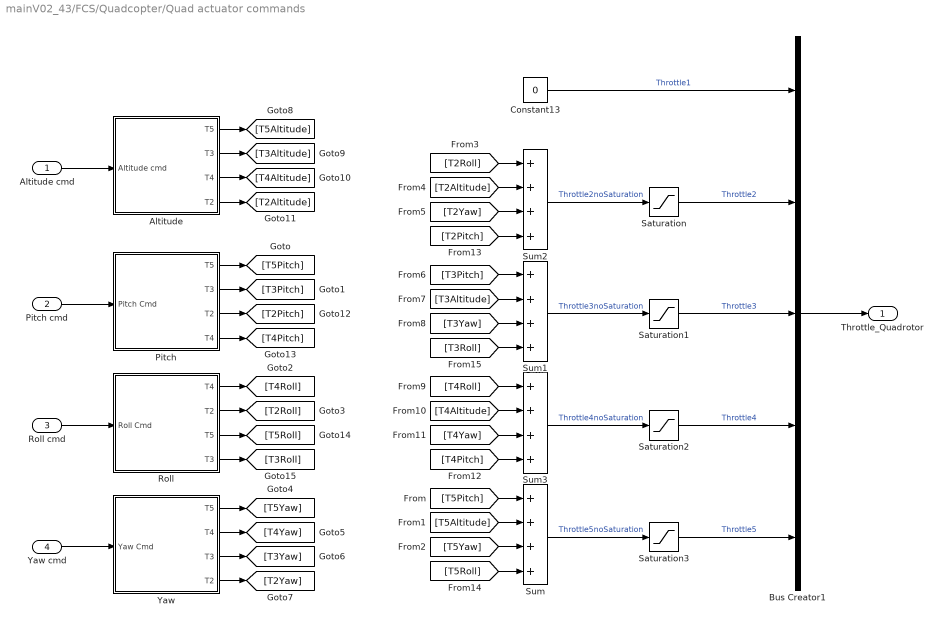
== system mainV02_43/FCS/Quadcopter/Quad actuator commands ==
  Altitude cmd : Inport
  Pitch cmd : Inport  Port=2
  Roll cmd : Inport  Port=3
  Yaw cmd : Inport  Port=4
  Altitude : Subsystem
  Bus Creator1 : BusCreator  Inputs='Throttle1','Throttle2','Throttle3','Throttle4','Throttle5'  OutDataTypeStr=Bus: ThrottleBus  NonVirtualBus=on
  Constant13 : Constant  Value=0
  Pitch : Subsystem
  Roll : Subsystem
  Saturation{,1..3} (4 alike) : Saturate  UpperLimit=1  LowerLimit=0
  Sum{,1..3} (4 alike) : Sum  Inputs=++++
  Yaw : Subsystem
  Throttle_Quadrotor : Outport  OutDataTypeStr=Bus: ThrottleBus
  wires:
  [T4Yaw] -> Sum3/3
  [T4Altitude] -> Sum3/2
  [T4Roll] -> Sum3/1
  [T3Yaw] -> Sum1/3
  [T3Altitude] -> Sum1/2
  [T3Pitch] -> Sum1/1
  [T2Yaw] -> Sum2/3
  [T2Altitude] -> Sum2/2
  [T2Roll] -> Sum2/1
  [T5Yaw] -> Sum/3
  [T5Altitude] -> Sum/2
  [T5Pitch] -> Sum/1
  Altitude/4(T2) -> [T2Altitude]
  Altitude/3(T4) -> [T4Altitude]
  Altitude/2(T3) -> [T3Altitude]
  Altitude/1(T5) -> [T5Altitude]
  Yaw/4(T2) -> [T2Yaw]
  Yaw/1(T5) -> [T5Yaw]
  Roll/2(T2) -> [T2Roll]
  Roll/1(T4) -> [T4Roll]
  Pitch/2(T3) -> [T3Pitch]
  Pitch/1(T5) -> [T5Pitch]
  Bus Creator1/1 -> Throttle_Quadrotor/1
  Pitch cmd/1 -> Pitch/1(Pitch Cmd)
  Roll cmd/1 -> Roll/1(Roll Cmd)
  Altitude cmd/1 -> Altitude/1(Altitude cmd)
  Yaw/2(T4) -> [T4Yaw]
  Yaw/3(T3) -> [T3Yaw]
  Yaw cmd/1 -> Yaw/1(Yaw Cmd)
  Pitch/3(T2) -> [T2Pitch]
  Pitch/4(T4) -> [T4Pitch]
  [T4Pitch] -> Sum3/4
  [T2Pitch] -> Sum2/4
  Roll/3(T5) -> [T5Roll]
  Roll/4(T3) -> [T3Roll]
  [T5Roll] -> Sum/4
  [T3Roll] -> Sum1/4
  Sum2/1 -> Saturation/1  "Throttle2noSaturation"
  Sum/1 -> Saturation3/1  "Throttle5noSaturation"
  Sum3/1 -> Saturation2/1  "Throttle4noSaturation"
  Sum1/1 -> Saturation1/1  "Throttle3noSaturation"
  Constant13/1 -> Bus Creator1/1  "Throttle1"
  Saturation/1 -> Bus Creator1/2  "Throttle2"
  Saturation1/1 -> Bus Creator1/3  "Throttle3"
  Saturation2/1 -> Bus Creator1/4  "Throttle4"
  Saturation3/1 -> Bus Creator1/5  "Throttle5"

== system mainV02_43/FCS/Quadcopter/Slider ==

== system mainV02_43/FCS/Quadcopter/Slider10 ==

== system mainV02_43/FCS/Quadcopter/Slider11 ==

== system mainV02_43/FCS/Quadcopter/Slider12 ==

== system mainV02_43/FCS/Quadcopter/Slider13 ==

== system mainV02_43/FCS/Quadcopter/Slider6 ==

== system mainV02_43/FCS/Quadcopter/Slider7 ==

== system mainV02_43/FCS/Quadcopter/Slider8 ==

== system mainV02_43/FCS/Quadcopter/Slider9 ==

== system mainV02_43/LIBIS Plant/Aerodynamics/CD ==
  prelook-ups : Inport
  plantData : Inport  Port=2
  actuators : Inport  Port=3
  Add : Sum  Inputs=+++++++
  Bus Selector : BusSelector  OutputSignals=alpha,alpha_dot,Omega_body.q
  Bus Selector1 : BusSelector  OutputSignals=alpha,beta,alt,xcg,deltae,deltar,deltafr,deltafl
  Bus Selector2 : BusSelector  OutputSignals=deltae,deltafr,deltafl
  CD0 : Interpolation_n-D  NumberOfTableDimensions=8  Table=LD.Stability.CD0  ExtrapMethod=Clip  DiagnosticForOutOfRangeInput=Warning  RequireIndexFractionAsBus=on  ValidIndexMayReachLast=on  InternalRulePriority=Speed
      settings: InputPortMap=u0,u1,u2,u3,u4,u5,u6,u7
  CDalpha : Interpolation_n-D  NumberOfTableDimensions=8  Table=LD.Stability.CDalpha  ExtrapMethod=Clip  DiagnosticForOutOfRangeInput=Warning  RequireIndexFractionAsBus=on  ValidIndexMayReachLast=on  InternalRulePriority=Speed
      settings: InputPortMap=u0,u1,u2,u3,u4,u5,u6,u7
  CDalpha_dot : Interpolation_n-D  NumberOfTableDimensions=8  Table=LD.Stability.CDalpha_dot  ExtrapMethod=Clip  RequireIndexFractionAsBus=on  ValidIndexMayReachLast=on  InternalRulePriority=Speed
      settings: InputPortMap=u0,u1,u2,u3,u4,u5,u6,u7
  CDdeltae : Interpolation_n-D  NumberOfTableDimensions=8  Table=LD.Stability.CDdeltae  ExtrapMethod=Clip  RequireIndexFractionAsBus=on  ValidIndexMayReachLast=on  InternalRulePriority=Speed
      settings: InputPortMap=u0,u1,u2,u3,u4,u5,u6,u7
  CDdeltafr : Interpolation_n-D  NumberOfTableDimensions=8  Table=LD.Stability.CDdeltafr  ExtrapMethod=Clip  RequireIndexFractionAsBus=on  ValidIndexMayReachLast=on  InternalRulePriority=Speed
      settings: InputPortMap=u0,u1,u2,u3,u4,u5,u6,u7
  CDdeltafrl : Interpolation_n-D  NumberOfTableDimensions=8  Table=LD.Stability.CDdeltafl  ExtrapMethod=Clip  RequireIndexFractionAsBus=on  ValidIndexMayReachLast=on  InternalRulePriority=Speed
      settings: InputPortMap=u0,u1,u2,u3,u4,u5,u6,u7
  CDq : Interpolation_n-D  NumberOfTableDimensions=8  Table=LD.Stability.CDq  ExtrapMethod=Clip  RequireIndexFractionAsBus=on  ValidIndexMayReachLast=on  InternalRulePriority=Speed
      settings: InputPortMap=u0,u1,u2,u3,u4,u5,u6,u7
  Product{,1..5} (6 alike) : Product
  CD : Outport
  wires:
  prelook-ups/1 -> Bus Selector1/1
  CD0/1 -> Add/1
  Add/1 -> CD/1
  plantData/1 -> Bus Selector/1
  actuators/1 -> Bus Selector2/1
  Product/1 -> Add/2
  Bus Selector/1 -> Product/2  "<alpha>"
  Bus Selector2/1 -> Product3/2  "<deltae>"
  CDdeltae/1 -> Product3/1
  Product3/1 -> Add/5
  Product2/1 -> Add/4
  Product1/1 -> Add/3
  CDalpha_dot/1 -> Product1/1
  CDq/1 -> Product2/1
  Bus Selector/3 -> Product2/2  "<q>"
  Bus Selector/2 -> Product1/2  "<alpha_dot>"
  Bus Selector1/8 -> CD0/8, CDalpha/8, CDq/8, CDdeltafrl/8, CDdeltafr/8, CDdeltae/8, CDalpha_dot/8  "<deltafl>"
  Bus Selector1/7 -> CD0/7, CDalpha/7, CDq/7, CDdeltafrl/7, CDdeltafr/7, CDdeltae/7, CDalpha_dot/7  "<deltafr>"
  Bus Selector1/6 -> CD0/6, CDalpha/6, CDq/6, CDdeltafrl/6, CDdeltafr/6, CDdeltae/6, CDalpha_dot/6  "<deltar>"
  Bus Selector1/5 -> CD0/5, CDalpha/5, CDq/5, CDdeltafrl/5, CDdeltafr/5, CDdeltae/5, CDalpha_dot/5  "<deltae>"
  Bus Selector1/3 -> CD0/3, CDalpha/3, CDq/3, CDdeltafrl/3, CDdeltafr/3, CDdeltae/3, CDalpha_dot/3  "<alt>"
  Bus Selector1/4 -> CD0/4, CDalpha/4, CDq/4, CDdeltafrl/4, CDdeltafr/4, CDdeltae/4, CDalpha_dot/4  "<xcg>"
  Bus Selector1/1 -> CD0/1, CDalpha/1, CDdeltafrl/1, CDdeltafr/1, CDdeltae/1, CDq/1, CDalpha_dot/1  "<alpha>"
  Bus Selector2/3 -> Product5/2  "<deltafl>"
  CDdeltafrl/1 -> Product5/1
  Product5/1 -> Add/7
  Product4/1 -> Add/6
  CDdeltafr/1 -> Product4/1
  Bus Selector2/2 -> Product4/2  "<deltafr>"
  Bus Selector1/2 -> CD0/2, CDdeltafrl/2, CDdeltafr/2, CDdeltae/2, CDq/2, CDalpha_dot/2, CDalpha/2  "<beta>"
  CDalpha/1 -> Product/1

== system mainV02_43/LIBIS Plant/Aerodynamics/CL ==
  prelook-ups : Inport
  plantData : Inport  Port=2
  actuators : Inport  Port=3
  Add1 : Sum  Inputs=+++++++
  Bus Selector2 : BusSelector  OutputSignals=alpha,alpha_dot,Omega_body.q
  Bus Selector4 : BusSelector  OutputSignals=alpha,beta,alt,xcg,deltae,deltar,deltafr,deltafl
  Bus Selector5 : BusSelector  OutputSignals=deltae,deltafr,deltafl
  CL0 : Interpolation_n-D  NumberOfTableDimensions=8  Table=LD.Stability.CL0  RequireIndexFractionAsBus=on  InternalRulePriority=Speed
      settings: InputPortMap=u0,u1,u2,u3,u4,u5,u6,u7
  CLalpha : Interpolation_n-D  NumberOfTableDimensions=8  Table=LD.Stability.CLalpha  ExtrapMethod=Clip  DiagnosticForOutOfRangeInput=Warning  RequireIndexFractionAsBus=on  ValidIndexMayReachLast=on  InternalRulePriority=Speed
      settings: InputPortMap=u0,u1,u2,u3,u4,u5,u6,u7
  CLalpha_dot : Interpolation_n-D  NumberOfTableDimensions=8  Table=LD.Stability.CLalpha_dot  ExtrapMethod=Clip  RequireIndexFractionAsBus=on  ValidIndexMayReachLast=on  InternalRulePriority=Speed
      settings: InputPortMap=u0,u1,u2,u3,u4,u5,u6,u7
  CLdeltae : Interpolation_n-D  NumberOfTableDimensions=8  Table=LD.Stability.CLdeltae  ExtrapMethod=Clip  RequireIndexFractionAsBus=on  ValidIndexMayReachLast=on  InternalRulePriority=Speed
      settings: InputPortMap=u0,u1,u2,u3,u4,u5,u6,u7
  CLdeltafr : Interpolation_n-D  NumberOfTableDimensions=8  Table=LD.Stability.CLdeltafr  ExtrapMethod=Clip  RequireIndexFractionAsBus=on  ValidIndexMayReachLast=on  InternalRulePriority=Speed
      settings: InputPortMap=u0,u1,u2,u3,u4,u5,u6,u7
  CLdeltafrl : Interpolation_n-D  NumberOfTableDimensions=8  Table=LD.Stability.CLdeltafl  ExtrapMethod=Clip  RequireIndexFractionAsBus=on  ValidIndexMayReachLast=on  InternalRulePriority=Speed
      settings: InputPortMap=u0,u1,u2,u3,u4,u5,u6,u7
  CLq : Interpolation_n-D  NumberOfTableDimensions=8  Table=LD.Stability.CLq  ExtrapMethod=Clip  RequireIndexFractionAsBus=on  ValidIndexMayReachLast=on  InternalRulePriority=Speed
      settings: InputPortMap=u0,u1,u2,u3,u4,u5,u6,u7
  Product{6..11} (6 alike) : Product
  CL : Outport
  wires:
  prelook-ups/1 -> Bus Selector4/1
  CL0/1 -> Add1/1
  Add1/1 -> CL/1
  plantData/1 -> Bus Selector2/1
  actuators/1 -> Bus Selector5/1
  Product6/1 -> Add1/2
  Bus Selector2/1 -> Product6/2  "<alpha>"
  Bus Selector5/1 -> Product9/2  "<deltae>"
  CLdeltae/1 -> Product9/1
  Product9/1 -> Add1/5
  Product8/1 -> Add1/4
  Product7/1 -> Add1/3
  CLalpha_dot/1 -> Product7/1
  CLq/1 -> Product8/1
  Bus Selector2/3 -> Product8/2  "<q>"
  Bus Selector2/2 -> Product7/2  "<alpha_dot>"
  Bus Selector4/8 -> CL0/8, CLalpha/8, CLq/8, CLdeltafrl/8, CLdeltafr/8, CLdeltae/8, CLalpha_dot/8  "<deltafl>"
  Bus Selector4/7 -> CL0/7, CLalpha/7, CLq/7, CLdeltafrl/7, CLdeltafr/7, CLdeltae/7, CLalpha_dot/7  "<deltafr>"
  Bus Selector4/6 -> CL0/6, CLalpha/6, CLq/6, CLdeltafrl/6, CLdeltafr/6, CLdeltae/6, CLalpha_dot/6  "<deltar>"
  Bus Selector4/5 -> CL0/5, CLalpha/5, CLq/5, CLdeltafrl/5, CLdeltafr/5, CLdeltae/5, CLalpha_dot/5  "<deltae>"
  Bus Selector4/3 -> CL0/3, CLalpha/3, CLq/3, CLdeltafrl/3, CLdeltafr/3, CLdeltae/3, CLalpha_dot/3  "<alt>"
  Bus Selector4/4 -> CL0/4, CLalpha/4, CLq/4, CLdeltafrl/4, CLdeltafr/4, CLdeltae/4, CLalpha_dot/4  "<xcg>"
  Bus Selector4/1 -> CL0/1, CLalpha/1, CLdeltafrl/1, CLdeltafr/1, CLdeltae/1, CLq/1, CLalpha_dot/1  "<alpha>"
  Bus Selector5/3 -> Product11/2  "<deltafl>"
  CLdeltafrl/1 -> Product11/1
  Product11/1 -> Add1/7
  Product10/1 -> Add1/6
  CLdeltafr/1 -> Product10/1
  Bus Selector5/2 -> Product10/2  "<deltafr>"
  Bus Selector4/2 -> CL0/2, CLdeltafrl/2, CLdeltafr/2, CLdeltae/2, CLq/2, CLalpha_dot/2, CLalpha/2  "<beta>"
  CLalpha/1 -> Product6/1

== system mainV02_43/LIBIS Plant/Aerodynamics/CY ==
  prelook-ups : Inport
  plantData : Inport  Port=2
  actuators : Inport  Port=3
  Add : Sum  Inputs=++++++
  Bus Selector : BusSelector  OutputSignals=beta,Omega_body.p,Omega_body.r
  Bus Selector1 : BusSelector  OutputSignals=alpha,beta,alt,xcg,deltae,deltar,deltafr,deltafl
  Bus Selector2 : BusSelector  OutputSignals=deltar,deltafr,deltafl
  CYbeta : Interpolation_n-D  NumberOfTableDimensions=8  Table=LD.Stability.CYbeta  ExtrapMethod=Clip  RequireIndexFractionAsBus=on  ValidIndexMayReachLast=on  InternalRulePriority=Speed
      settings: InputPortMap=u0,u1,u2,u3,u4,u5,u6,u7
  CYdeltafl : Interpolation_n-D  NumberOfTableDimensions=8  Table=LD.Stability.CYdeltafl  ExtrapMethod=Clip  RequireIndexFractionAsBus=on  ValidIndexMayReachLast=on  InternalRulePriority=Speed
      settings: InputPortMap=u0,u1,u2,u3,u4,u5,u6,u7
  CYdeltafr : Interpolation_n-D  NumberOfTableDimensions=8  Table=LD.Stability.CYdeltafr  ExtrapMethod=Clip  RequireIndexFractionAsBus=on  ValidIndexMayReachLast=on  InternalRulePriority=Speed
      settings: InputPortMap=u0,u1,u2,u3,u4,u5,u6,u7
  "CYdeltar " : Interpolation_n-D  NumberOfTableDimensions=8  Table=LD.Stability.CYdeltar  ExtrapMethod=Clip  RequireIndexFractionAsBus=on  ValidIndexMayReachLast=on  InternalRulePriority=Speed
      settings: InputPortMap=u0,u1,u2,u3,u4,u5,u6,u7
  CYp : Interpolation_n-D  NumberOfTableDimensions=8  Table=LD.Stability.CYp  ExtrapMethod=Clip  RequireIndexFractionAsBus=on  ValidIndexMayReachLast=on  InternalRulePriority=Speed
      settings: InputPortMap=u0,u1,u2,u3,u4,u5,u6,u7
  CYr : Interpolation_n-D  NumberOfTableDimensions=8  Table=LD.Stability.CYr  ExtrapMethod=Clip  RequireIndexFractionAsBus=on  ValidIndexMayReachLast=on  InternalRulePriority=Speed
      settings: InputPortMap=u0,u1,u2,u3,u4,u5,u6,u7
  Product{,1..5} (6 alike) : Product
  CY : Outport
  wires:
  Bus Selector1/8 -> CYbeta/8, CYr/8, "CYdeltar "/8, CYdeltafl/8, CYdeltafr/8, CYp/8  "<deltafl>"
  Bus Selector1/7 -> CYbeta/7, CYr/7, "CYdeltar "/7, CYdeltafl/7, CYdeltafr/7, CYp/7  "<deltafr>"
  Bus Selector1/6 -> CYbeta/6, CYr/6, "CYdeltar "/6, CYdeltafl/6, CYdeltafr/6, CYp/6  "<deltar>"
  prelook-ups/1 -> Bus Selector1/1
  Bus Selector1/5 -> CYbeta/5, CYr/5, "CYdeltar "/5, CYdeltafl/5, CYdeltafr/5, CYp/5  "<deltae>"
  Bus Selector1/3 -> CYbeta/3, CYr/3, "CYdeltar "/3, CYdeltafl/3, CYdeltafr/3, CYp/3  "<alt>"
  Bus Selector1/4 -> CYbeta/4, CYr/4, "CYdeltar "/4, CYdeltafl/4, CYdeltafr/4, CYp/4  "<xcg>"
  Bus Selector1/1 -> CYbeta/1, CYdeltafl/1, CYdeltafr/1, "CYdeltar "/1, CYr/1, CYp/1  "<alpha>"
  Add/1 -> CY/1
  plantData/1 -> Bus Selector/1
  actuators/1 -> Bus Selector2/1
  CYbeta/1 -> Product/1
  Product/1 -> Add/1
  Bus Selector/1 -> Product/2  "<beta>"
  Bus Selector2/1 -> Product3/2  "<deltar>"
  "CYdeltar "/1 -> Product3/1
  Product3/1 -> Add/4
  Product2/1 -> Add/3
  Product1/1 -> Add/2
  CYp/1 -> Product1/1
  CYr/1 -> Product2/1
  Bus Selector/3 -> Product2/2  "<r>"
  Bus Selector/2 -> Product1/2  "<p>"
  CYdeltafl/1 -> Product5/1
  Product5/1 -> Add/6
  Product4/1 -> Add/5
  CYdeltafr/1 -> Product4/1
  Bus Selector2/2 -> Product4/2  "<deltafr>"
  Bus Selector2/3 -> Product5/2  "<deltafl>"
  Bus Selector1/2 -> CYdeltafl/2, CYdeltafr/2, "CYdeltar "/2, CYr/2, CYp/2, CYbeta/2  "<beta>"

== system mainV02_43/LIBIS Plant/Aerodynamics/Cl ==
  prelook-ups1 : Inport
  plantData : Inport  Port=2
  actuators : Inport  Port=3
  Add1 : Sum  Inputs=++++++
  Bus Selector3 : BusSelector  OutputSignals=beta,Omega_body.p,Omega_body.r
  Bus Selector4 : BusSelector  OutputSignals=alpha,beta,alt,xcg,deltae,deltar,deltafr,deltafl
  Bus Selector5 : BusSelector  OutputSignals=deltar,deltafr,deltafl
  Clbeta : Interpolation_n-D  NumberOfTableDimensions=8  Table=LD.Stability.Clbeta  ExtrapMethod=Clip  RequireIndexFractionAsBus=on  ValidIndexMayReachLast=on  InternalRulePriority=Speed
      settings: InputPortMap=u0,u1,u2,u3,u4,u5,u6,u7
  Cldeltafl : Interpolation_n-D  NumberOfTableDimensions=8  Table=LD.Stability.Cldeltafl  ExtrapMethod=Clip  RequireIndexFractionAsBus=on  ValidIndexMayReachLast=on  InternalRulePriority=Speed
      settings: InputPortMap=u0,u1,u2,u3,u4,u5,u6,u7
  Cldeltafr : Interpolation_n-D  NumberOfTableDimensions=8  Table=LD.Stability.Cldeltafr  ExtrapMethod=Clip  RequireIndexFractionAsBus=on  ValidIndexMayReachLast=on  InternalRulePriority=Speed
      settings: InputPortMap=u0,u1,u2,u3,u4,u5,u6,u7
  "Cldeltar " : Interpolation_n-D  NumberOfTableDimensions=8  Table=LD.Stability.Cldeltar  ExtrapMethod=Clip  RequireIndexFractionAsBus=on  ValidIndexMayReachLast=on  InternalRulePriority=Speed
      settings: InputPortMap=u0,u1,u2,u3,u4,u5,u6,u7
  Clp : Interpolation_n-D  NumberOfTableDimensions=8  Table=LD.Stability.Clp  ExtrapMethod=Clip  RequireIndexFractionAsBus=on  ValidIndexMayReachLast=on  InternalRulePriority=Speed
      settings: InputPortMap=u0,u1,u2,u3,u4,u5,u6,u7
  Clr : Interpolation_n-D  NumberOfTableDimensions=8  Table=LD.Stability.Clr  ExtrapMethod=Clip  RequireIndexFractionAsBus=on  ValidIndexMayReachLast=on  InternalRulePriority=Speed
      settings: InputPortMap=u0,u1,u2,u3,u4,u5,u6,u7
  Product{6..11} (6 alike) : Product
  Cl : Outport
  wires:
  Bus Selector4/8 -> Clbeta/8, Clr/8, "Cldeltar "/8, Cldeltafl/8, Cldeltafr/8, Clp/8  "<deltafl>"
  Bus Selector4/7 -> Clbeta/7, Clr/7, "Cldeltar "/7, Cldeltafl/7, Cldeltafr/7, Clp/7  "<deltafr>"
  Bus Selector4/6 -> Clbeta/6, Clr/6, "Cldeltar "/6, Cldeltafl/6, Cldeltafr/6, Clp/6  "<deltar>"
  prelook-ups1/1 -> Bus Selector4/1
  Bus Selector4/5 -> Clbeta/5, Clr/5, "Cldeltar "/5, Cldeltafl/5, Cldeltafr/5, Clp/5  "<deltae>"
  Bus Selector4/3 -> Clbeta/3, Clr/3, "Cldeltar "/3, Cldeltafl/3, Cldeltafr/3, Clp/3  "<alt>"
  Bus Selector4/4 -> Clbeta/4, Clr/4, "Cldeltar "/4, Cldeltafl/4, Cldeltafr/4, Clp/4  "<xcg>"
  Bus Selector4/1 -> Clbeta/1, Cldeltafl/1, Cldeltafr/1, "Cldeltar "/1, Clr/1, Clp/1  "<alpha>"
  Add1/1 -> Cl/1
  plantData/1 -> Bus Selector3/1
  actuators/1 -> Bus Selector5/1
  Clbeta/1 -> Product6/1
  Product6/1 -> Add1/1
  Bus Selector3/1 -> Product6/2  "<beta>"
  Bus Selector5/1 -> Product9/2  "<deltar>"
  "Cldeltar "/1 -> Product9/1
  Product9/1 -> Add1/4
  Product8/1 -> Add1/3
  Product7/1 -> Add1/2
  Clp/1 -> Product7/1
  Clr/1 -> Product8/1
  Bus Selector3/3 -> Product8/2  "<r>"
  Bus Selector3/2 -> Product7/2  "<p>"
  Cldeltafl/1 -> Product11/1
  Product11/1 -> Add1/6
  Product10/1 -> Add1/5
  Cldeltafr/1 -> Product10/1
  Bus Selector5/2 -> Product10/2  "<deltafr>"
  Bus Selector5/3 -> Product11/2  "<deltafl>"
  Bus Selector4/2 -> Cldeltafl/2, Cldeltafr/2, "Cldeltar "/2, Clr/2, Clp/2, Clbeta/2  "<beta>"
